simulink model "main_sim_noadapt"  (Simulink 7.2)
settings: Solver=ode2  SolverMode=SingleTasking  StartTime=0.0  StopTime=tsim_max  FixedStep=dtsim  RelTol=1e-3
StopFcn:
  | %mkplt
values from neighbouring files (symbols this model uses):
  vel = 128    [do_command_tracking.m]
undefined symbols (not defined in the file or in its folder): accel_cmd, aero_surf_qbar_off, aero_surf_qbar_on, assertion_time, att_cmd_select, att_trim_IC, att_type, att_type_numbers, bb_ellipsoid, bb_params, chi_trim_IC, command_time, compute_all_rate_cols, compute_all_vel_cols, constants, cosA, da_trim_IC, dc_L2W_IC, de_trim_IC, DiscIntNeverNeededParam, dr_trim_IC, dtsim, E_rwy, E_trim_IC, Ed_cmd, Ed_trim_IC, eow_boundary, flag_exsig, full_surf_llim, full_surf_ulim, gain_set, gain_var_struct, gam_cmd_descent, gam_cmd_preflare, gamdot_cmd_descent, gamdot_cmd_flare, gamdot_cmd_preflare, gamma_trim_IC, h_trim_IC, hd_cmd, hd_trim_IC, ideal_vel_Kb, in_exsig_vecin, in_exsig_vecout, in_t_exsig, MACH, MACH_att_fb, MACH_att_int_IC, MACH_att_Kb, MACH_att_Kc, MACH_att_Ki, MACH_gain_mat, MACH_mass_IC, MACH_pos_IC, MACH_pos_int_IC, MACH_pos_Kb, MACH_pos_Kc, MACH_pos_Ki, MACH_pqr_Bmat_IC, MACH_pqr_IC ... (+62)
libraries: simulink x36, utility_lib x34, mach_lib x24, model_lib x13, simulink_need_slupdate x8, models x8
(part 7 of 7)

== matlab function claw_main/rate_loops/bangbang/Bang Bang ==
  data: bb_params input double; bb_ellipsoid input double; debug_output output double; cvddes output double; dir output double; use_bb output double; att_cvc input double; att_cv input double; timer output double; pqr input double; inertia input double; enable_bb input double; cvddes_lin input double; dir_old input double; use_bb_old input double; timer_old input double
function [debug_output,cvddes,dir,use_bb,timer] = bangbang(bb_params,bb_ellipsoid,att_cvc,att_cv,pqr,inertia,enable_bb,cvddes_lin,dir_old,use_bb_old,timer_old)
% This block supports an embeddable subset of the MATLAB language.
% See the help menu for details. 

dt = bb_params(1) ;
timer_max = bb_params(2) ;
att_thresh = bb_params(3) ;
rate_thresh = bb_params(4) ;
att_diff_thresh = bb_params(5) ;
pp_params = bb_params(6:end) ;

debug_output = zeros(12,1) ;
cvddes = cvddes_lin ;
use_bb = 0 ;
dir = zeros(3,1) ;
timer = timer_old ;

if( ~enable_bb )
    return
end
    
trans = qmpy([1 -1 -1 -1]'.*att_cv,att_cvc) ;

% default is to use dir_old if we were in bangbang last cycle,
% and the timer has not expired
use_dir_old = use_bb_old ;
if( use_dir_old )
    timer = timer + dt ;
    if( timer > timer_max )
        % if timer expires, don't use dir_old
        use_dir_old = 0 ;
    end
end

% compute att using current transformation quat
trans_mag = trans(1) ;
trans_dir = trans(2:4) ;
att = -2*atan2(norm_vec3(trans_dir),trans_mag) ;
att_old = -2*atan2(dir_old'*trans_dir,trans_mag) ;

% choose arbitrary att (and dir) sign to be the same as that computed using
% dir_old.  This is equivalent to making dir_old'*trans_dir positive.
if( att*att_old < 0 )
    att = -att ;
    trans_dir = -trans_dir ;
end

% if we intended to use dir_old, but the angle computed using
% dir_old is significantly different than that derived using the current
% transformation, we will use current dir.
% NOTE: the angle test below works only because att has been adjusted
% to have the same sign as att_old, and both result from atan2 
if( use_dir_old )
    if( abs(att - att_old) > att_diff_thresh )
        use_dir_old = 0 ;
    else
        dir = dir_old ;
        att = att_old ;
    end
end

% check condition to enter (or stay in) bangbang
if( abs(att) > att_thresh )
    use_bb = 1 ;
    
    if( ~use_dir_old )
        dir = trans_dir/norm_vec3(trans_dir) ;
        timer = 0 ;
    end

elseif( max(abs(pqr)) > rate_thresh )
    use_bb = 1 ;
    
    % if small attitude error, set dir based on rates
    if( ~use_dir_old )
        dir = pqr/norm_vec3(pqr) ;
        att = -2*atan2(dir'*trans_dir,trans_mag) ;
        timer = 0 ;
    end
else
    % even though not used, pass dir_old through for in case of ~use_bb
    dir = dir_old ;
    att = att_old ;
end

% Note: cvddes has been set to a default value of cvddes_lin

if( use_bb )
    rate = pqr'*dir ;
    accel_max = get_ellipsoid_scaling(inertia*dir,bb_ellipsoid) ;
    accel_min = -accel_max ;
    pp_params(1) = accel_max ;
    pp_params(2) = accel_min ;
    [outside,accel] = pp(pp_params,att,rate) ;
    
    if( outside <= 1 )
        % use default cvddes (cvddes_lin)
        use_bb = 0 ; 
    else
        % eliminate component of linear command in direction dir
        cvddes = cvddes - (dir'*cvddes)*dir ;
    end
else
    % use default cvddes (cvddes_lin)
    rate = 0 ;
    outside = 0 ;
    accel = 0 ;
end

% saturate command at ellipsoid
blend_lin_claw = cvddes*min(get_ellipsoid_scaling(inertia*cvddes,bb_ellipsoid),1) ;

% add component from bangbang
blend_bb_claw = accel*dir ;
cvddes = blend_lin_claw + blend_bb_claw ;

pp_utQu = 1/get_ellipsoid_scaling(inertia*cvddes,bb_ellipsoid) ;
debug_output = [att;att_old;rate;outside;accel;pp_utQu;blend_bb_claw;blend_lin_claw] ;

if( ~use_bb )
    
    % if not using bangbang reset the timer, and set dir to zero
    timer = 0 ;
    % dir used for cvd_des blending is now zeroed outside of this block,
    % so that dir can be retained through a temporary ~use_bb condition
%     dir = 0*dir ;
end

function r = qmpy(p,q)

p0 = p(1) ;
p1 = p(2) ;
p2 = p(3) ;
p3 = p(4) ;

q0 = q(1) ;
q1 = q(2) ;
q2 = q(3) ;
q3 = q(4) ;

r0 = p0 * q0 - p1 * q1 - p2 * q2 - p3 * q3 ;
r1 = p0 * q1 + p1 * q0 + p2 * q3 - p3 * q2 ;
r2 = p0 * q2 - p1 * q3 + p2 * q0 + p3 * q1 ;
r3 = p0 * q3 + p1 * q2 - p2 * q1 + p3 * q0 ;

r = [ r0 r1 r2 r3 ]' ;

function scale = get_ellipsoid_scaling(dir,ellipsoid)
    scale = 1/max(sqrt(dir'*(ellipsoid*dir)),1e-12) ;

function [outside,accel] = pp(params,att,rate)

% the linear control law is
% accel = ww^2 * ( att_cmd - att ) - 2 * zeta * ww * rate

amax = params(1) ; 
amin = params(2) ; 
ww = params(3) ;  
zeta = params(4) ; 
rate_des1 = params(5) ; 
rate_des2 = params(6) ;

% make switch curves conservative
swcurve_shrink = 1.0 ;

swcurve_pos = 0.5 * rate^2 - swcurve_shrink * amin * att ;
swcurve_neg = 0.5 * rate^2 - swcurve_shrink * amax * att ;

% replace ellipse with parallelogram
% outside = ( ww^2 * att^2 + 2 * zeta * ww * att * rate + rate^2 ) / ( ( 1 - zeta^2 ) * amax^2 / ww^2 ) ;
sx1 = 1 + zeta + 4 * zeta^2 ;
sv1 = -0.5 - 2 * zeta ;
sx2 = 1 - 4 * zeta^2
sv2 = 2 * zeta ;
p1 = [sx1; sv1] ;
p2 = [sx2; sv2] ;

outside = 2*ww/amax*max(abs(([p2+p1 p2-p1]\[att*ww; rate])))
accel = 0 ;

if( outside <= 1 )
    return
end

if( rate > 0 )
    if( swcurve_pos < 0 )
        if( rate < rate_des1 )
            accel = amax ;
        elseif( rate < rate_des2 )
            accel = 0 ;
        else
            accel = amin ;
        end
    else
        accel = amin ;
    end
else
    if( swcurve_neg < 0 )
        if( rate > -rate_des1 )
            accel = amin ;
        elseif( rate > - rate_des2 )
            accel = 0 ;
        else
            accel = amax ;
        end
    else
        accel = amax ;
    end
end


function out = norm_vec3(in)

out = sqrt(in(1)^2 + in(2)^2 + in(3)^2);

return
